simulink model "proj_liion"  (R2021a)
settings: Solver=VariableStepAuto  StartTime=0.0  StopTime=1000  RelTol=1e-3
undefined symbols (not defined in the file): Ion, Lithium
libraries: spsSeriesRLCBranchLib x4, spsDiodeLib x4, spsCurrentMeasurementLib x2, spsMeanLib x2, spsMosfetLib x2, spsVoltageMeasurementLib x2, spsVariableResistorLib x2, spsACVoltageSourceLib x1, spsBatteryLib x1, spsGroundLib x1, spspowerguiLib x1
settings Model: Creator=Hxtreme  LastModifiedBy=ARULARASU

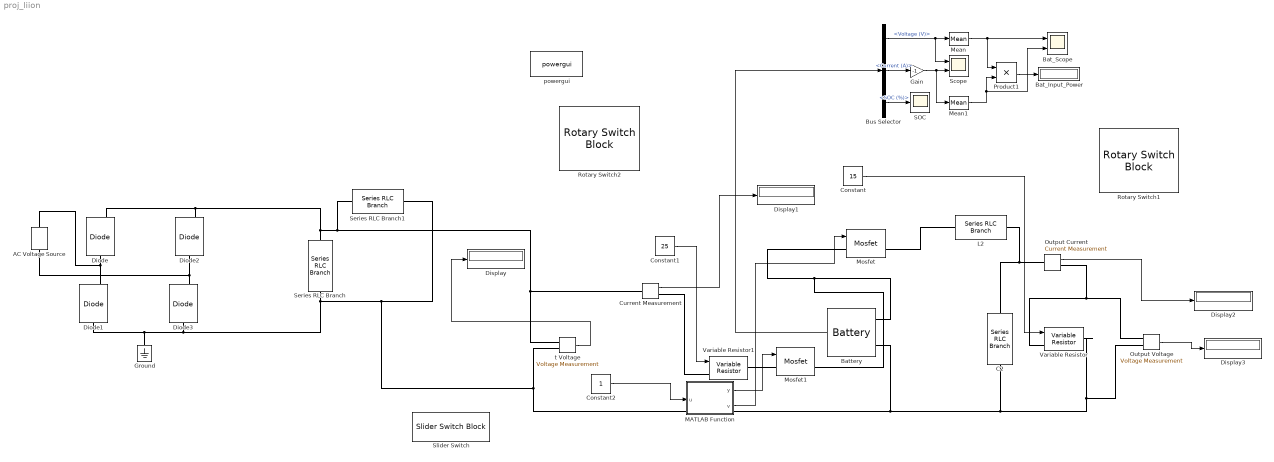
== system proj_liion ==
  AC Voltage Source : spsACVoltageSourceLib/AC Voltage Source  Amplitude=220  Phase=0  Frequency=60  SampleTime=0  Measurements=None  BusType=swing  Pref=10e3  Qref=0  Qmin=-inf  Qmax=+inf
  Bat_Input_Power : Display
  Bat_Scope : Scope  NumInputPorts=2
  Battery : spsBatteryLib/Battery  BatType=Lithium-Ion  ShowTempParam=off  ThermalPreset=no  ShowAgeParam=off  NomV=48  NomQ=2  SOC=100  Batt_Tr=30  PresetModel=on  MaxQ=2  MinV=36  FullV=55.8714  Dis_rate=0.86957  R=0.24  Normal_OP=1.8087  expZone="[51.8585    0.0982609]"  current=[6.5 13 32.5]  Units=Time  Tci=20  NomT=20  T2=-30  MaxQ2=4.8  FullV2=7.1  Normal_OP2=5.655  expZone2="[6.58           1]"  Rca=0.6  ti=2000  Dp=0  Neq0=0  Tsim=1e6  Ta1=25  Qeol=5.4*0.9  Reol=0.013333*1.2  Char_age=[2.3478, 3]  Dis_age=[2.3478, 10]  N1=1500  N2=10500  N3=1000  N4=1400  Ta2=45  N5=950
  Bus Selector : BusSelector  OutputSignals=Voltage (V),Current (A),SOC (%)
  C2 : spsSeriesRLCBranchLib/Series RLC Branch  LConnTagsString=__new0  RConnTagsString=__new0  BranchType=C  Resistance=1  Inductance=1e-3  SetiL0=off  InitialCurrent=0  Capacitance=3.33e-6  Setx0=off  InitialVoltage=0  Measurements=None
  Constant : Constant  Value=15
  Constant1 : Constant  Value=25
  Constant2 : Constant
  Current Measurement : spsCurrentMeasurementLib/Current Measurement  PhasorSimulation=off  OutputType=Complex  PSBequivalent=0
  Diode{,1..3} (4 alike) : spsDiodeLib/Diode  Ron=0.001  Lon=0  Vf=0.8  IC=0  UseSnubber=0  Rs=500  Cs=250e-9  Measurements=on
  Display{,1..3} (4 alike) : Display
  Gain : Gain  Gain=-1
  Ground : spsGroundLib/Ground  LConnTagsString=a
  L2 : spsSeriesRLCBranchLib/Series RLC Branch  LConnTagsString=__new0  RConnTagsString=__new0  BranchType=L  Resistance=1  Inductance=681e-6  SetiL0=off  InitialCurrent=0  Capacitance=1e-6  Setx0=off  InitialVoltage=0  Measurements=None
  MATLAB Function : MATLAB Function  TreatAsAtomicUnit=on
  Mean : spsMeanLib/Mean  Freq=50  Vinit=0  Ts=0
  Mean1 : spsMeanLib/Mean  Freq=50  Vinit=0  Ts=0
  Mosfet : spsMosfetLib/Mosfet  Ron=0.1  Lon=0  Rd=0.01  Vfd=0  IC=0  Rs=1e5  Cs=inf  Measurements=on
  Mosfet1 : spsMosfetLib/Mosfet  Ron=0.1  Lon=0  Rd=0.01  Vfd=0  IC=0  Rs=1e5  Cs=inf  Measurements=on
  "Output Current " : spsCurrentMeasurementLib/Current Measurement  PhasorSimulation=off  OutputType=Complex  PSBequivalent=0
  Output Voltage : spsVoltageMeasurementLib/Voltage Measurement  PhasorSimulation=off  OutputType=Complex  PSBequivalent=0
  Product1 : Product
  Rotary Switch1 : RotarySwitchBlock
      settings: Values={{'No Load', 'Load 1', 'Load 2', 'Load 3'}, [10 15 20 25]}
  Rotary Switch2 : RotarySwitchBlock
      settings: Values={{'No Load', 'Load 1', 'Load 2', 'Load 3'}, [10 15 20 25]}
  SOC : Scope
  Scope : Scope  NumInputPorts=2
  Series RLC Branch : spsSeriesRLCBranchLib/Series RLC Branch  LConnTagsString=__new0  RConnTagsString=__new0  BranchType=R  Resistance=10000  Inductance=1e-3  SetiL0=off  InitialCurrent=0  Capacitance=1e-6  Setx0=off  InitialVoltage=0  Measurements=None
  Series RLC Branch1 : spsSeriesRLCBranchLib/Series RLC Branch  LConnTagsString=__new0  RConnTagsString=__new0  BranchType=C  Resistance=1  Inductance=1e-3  SetiL0=off  InitialCurrent=0  Capacitance=1000e-6  Setx0=off  InitialVoltage=0  Measurements=None
  Slider Switch : SliderSwitchBlock
      settings: Values={{'Off', 'On'}, [1 2]}
  Variable Resistor : spsVariableResistorLib/Variable Resistor  Rabsmin=1e-3
      settings: SourceProductBaseCode=PS
  Variable Resistor1 : spsVariableResistorLib/Variable Resistor  Rabsmin=1e-3
      settings: SourceProductBaseCode=PS
  powergui : spspowerguiLib/powergui  Priority=1  SimulationMode=Discrete  SampleTime=1e-5  frequency=60  Iterations=50  frequencyindice=0  Pbase=100e6  ErrMax=1e-4  UnitsV=kV  UnitsW=MW  buscounter=0  FunctionMessages=off  echomessages=off  EnableUseOfTLC=off  CurrentSourceSwitches=off  DisableSnubberDevices=off  DisableRonSwitches=off  DisableVfSwitches=off  DisplayEquations=off  AutomaticDiscreteSolvers=off  SolverType=Tustin/Backward Euler (TBE)  Interpol=off  ExternalGateDelay=off  methode=off  Ts=100  x0status=blocks  SPID=on  SwTol=0  HookPort=off  NonlinearTolerance=1e-4  nMaxIteration=100  ContinueOnMaxIteration=off  RestoreLinks=warning  ResistiveCurrentMeasurement=off  Frange=[0:2:500]  Ylog=off  Xlog=on  ShowGrid=off  save=off  variable=ZData  structure=0  ZoomFFT=off  StartTime=0.0  cycles=1  DisplayStyle=1  fundamental=60  FreqAxis=off  MaxFrequency=1000  frequencyindicesteady=1  RmsSteady=1  display=off
  t Voltage : spsVoltageMeasurementLib/Voltage Measurement  PhasorSimulation=off  OutputType=Complex  PSBequivalent=0
  wires:
  t Voltage/1 -> Display/1
  Current Measurement/1 -> Display1/1
  "Output Current "/1 -> Display2/1
  Output Voltage/1 -> Display3/1
  Constant/1 -> Variable Resistor/1
  Constant1/1 -> Variable Resistor1/1
  Product1/1 -> Bat_Input_Power/1
  Mean/1 -> Bat_Scope/1, Product1/1
  Bus Selector/2 -> Gain/1  "<Current (A)>"
  Mean1/1 -> Bat_Scope/2, Product1/2
  Battery/1 -> Bus Selector/1
  Bus Selector/1 -> Scope/1, Mean/1  "<Voltage (V)>"
  Gain/1 -> Mean1/1, Scope/2
  Bus Selector/3 -> SOC/1  "<SOC (%)>"
  Constant2/1 -> MATLAB Function/1(u)
  MATLAB Function/1(y) -> Mosfet1/1
  MATLAB Function/2(v) -> Mosfet/1
  connections:
  Ground/LConn1 -- Diode1/LConn1 -- Diode3/LConn1 -- Series RLC Branch1/RConn1 -- Variable Resistor/RConn1 -- Output Voltage/LConn2 -- C2/RConn1 -- Battery/LConn2 -- t Voltage/LConn2 -- Series RLC Branch/RConn1
  "Output Current "/LConn1 -- C2/LConn1 -- L2/RConn1
  "Output Current "/RConn1 -- Variable Resistor/LConn1 -- Output Voltage/LConn1
  Mosfet/LConn1 -- Mosfet1/RConn1 -- Battery/LConn1
  Current Measurement/RConn1 -- Variable Resistor1/LConn1
  Diode1/RConn1 -- Diode/LConn1 -- AC Voltage Source/RConn1
  Diode3/RConn1 -- Diode2/LConn1 -- AC Voltage Source/LConn1
  t Voltage/LConn1 -- Current Measurement/LConn1 -- Series RLC Branch1/LConn1 -- Series RLC Branch/LConn1 -- Diode/RConn1 -- Diode2/RConn1
  Mosfet/RConn1 -- L2/LConn1
  Mosfet1/LConn1 -- Variable Resistor1/RConn1

== matlab function proj_liion/MATLAB Function ==
  data: u input; y output; v output
function [y,v]= fcn(u)
v=0;
y=0;
if u==1
    y=1;
    v=0;
elseif u==2
    v=1;
    y=0;
end
